simulink model "model"  (R2021b)
settings: Solver=VariableStepAuto  StartTime=0.0  StopTime=10.0  RelTol=1e-3
undefined symbols (not defined in the file): Newton, Raphson
settings Model: Creator=O  LastModifiedBy=ojiken

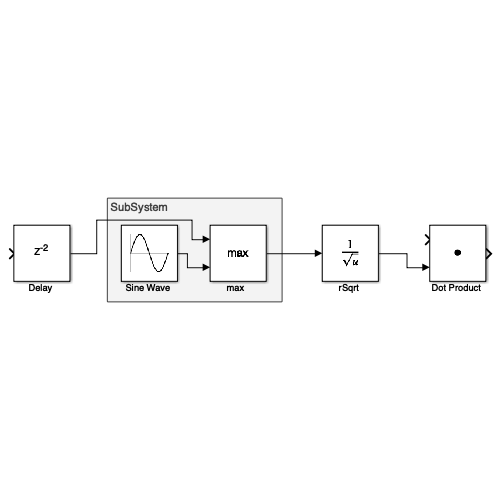
[thumbnail: Simulink's stored preview of the top-level diagram]
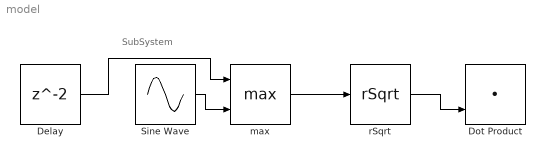
== system model ==
  note: SubSystem
  "Delay " : Delay  SampleTime=1
  "Dot Product " : DotProduct  OutDataTypeStr=double  InputSameDT=on
  "Sine Wave " : Sin  Amplitude=[-506831533.045897]  Bias=[-374132303.029973]  SampleTime=0
  "max  " : MinMax  Function=max  Inputs=2  OutDataTypeStr=double
  "rSqrt " : Sqrt  Operator=rSqrt  OutDataTypeStr=double  AlgorithmType=Newton-Raphson  SaturateOnIntegerOverflow=on
  wires:
  "Sine Wave "/1 -> "max  "/2
  "rSqrt "/1 -> "Dot Product "/2
  "max  "/1 -> "rSqrt "/1
  "Delay "/1 -> "max  "/1
